simulink model "gdnn_lm_rtrl"  (R2017b)
settings: Solver=ode5  StartTime=0.0  StopTime=train_length  FixedStep=T_sim  RelTol=1e-3  EnableMultiTasking=on
values from neighbouring files (symbols this model uses):
  bb = zeros(1,numoflayers)    [ini_gdnn.m]
  bs = zeros(1,numoflayers)    [ini_gdnn.m]
  D_max = max(max(max(max(idel))),max(max(max(ldel))))    [ini_gdnn.m]
  DI_vec = [DI_vec DI(i,:)]    [ini_gdnn.m]
  DIB_vec = [DIB_vec DIB(i,:)]    [ini_gdnn.m]
  dimax = max(dimax)    [ini_gdnn.m]
  DIS_vec = [DIS_vec DIS(i,:)]    [ini_gdnn.m]
  DL_vec = [DL_vec DL(i,:)]    [ini_gdnn.m]
  DLB_vec = [DLB_vec DLB(i,:)]    [ini_gdnn.m]
  dlmax = max(dlmax)    [ini_gdnn.m]
  DLS_vec = [DLS_vec DLS(i,:)]    [ini_gdnn.m]
  E_LW_U = zeros(1,numoflayers^2)    [ini_gdnn.m]
  I = zeros(1,numoflayers*numofinputs)    [ini_gdnn.m]
  idelb_vec = 0    [ini_gdnn.m]
  idels_vec = 0    [ini_gdnn.m]
  Lb = zeros(1,numoflayers^2)    [ini_gdnn.m]
  ldelb_vec = 0    [ini_gdnn.m]
  ldels_vec = 0    [ini_gdnn.m]
  Lf = zeros(1,numoflayers^2)    [ini_gdnn.m]
  net_params = [Q, mue, theta, T, L, D_max, numoflayers, numofinputs, max(S), sum(R), S_out, S_target, print_weights, min_weights, prune_interval, train_length, prune_maxerr_OBS, prune_maxerr_exact]    [ini_gdnn.m]
  Q = 500    [ini_gdnn.m]
  T = 0.01    [APRBS_Anregung_APRBS.m]    (also in ini_gdnn.m)
  U = U_target    [ini_gdnn.m]
  U_out = zeros(1,numoflayers)    [ini_gdnn.m]
  U_target = zeros(1,numoflayers)    [ini_gdnn.m]
  W_alpha_ini = ones(1,L)    [ini_gdnn.m]
  W_ini = rand(1,L) - 0.5    [ini_gdnn.m]
  X = zeros(1,numoflayers)    [ini_gdnn.m]
undefined symbols (not defined in the file or in its folder): idel_vec, ldel_vec, R, S
libraries: mblibv1 x13, simulink x3
CloseFcn:
  | rtwprivate ssgencode ModelCloseRequest gdnn_lm_rtrl
settings Model: Creator=endisch  LastModifiedBy=Ussaema
settings DataIOCC: LimitDataPoints=on  SaveFormat=Array  SignalLoggingSaveFormat=ModelDataLogs
settings OptimizationCC: InitFltsAndDblsToZero=on  LifeSpan=inf
settings DebuggingCC: SaveWithParameterizedLinksMsg=none  UnderspecifiedInitializationDetection=Classic  MergeDetectMultiDrivingBlocksExec=none  SignalResolutionControl=TryResolveAllWithWarning  SolverPrmCheckMsg=warning  MultiTaskDSMMsg=warning  MultiTaskCondExecSysMsg=none  FcnCallInpInsideContextMsg=warning  StateNameClashWarn=warning  StrictBusMsg=None  SFUnexpectedBacktrackingDiag=warning  SFNoUnconditionalDefaultTransitionDiag=warning  SFExecutionAtInitializationDiag=none
settings HardwareCC: ProdBitPerPointer=32  ProdBitPerSizeT=32  ProdBitPerPtrDiffT=32  ProdLargestAtomicFloat=None  ProdIntDivRoundTo=Undefined  ProdEndianess=Unspecified  ProdWordSize=32  ProdHWDeviceType=32-bit Generic
settings ModelReferenceCC: PropagateSignalLabelsOutOfModel=off
settings CodeAppCC: StateflowObjectComments=on
settings GRTTargetCC: TargetFcnLib=ansi_tfl_tmw.mat  TargetLangStandard=C89/C90 (ANSI)  GeneratePreprocessorConditionals=Disable all  CombineOutputUpdateFcns=off  GRTInterface=on
settings ConfigComp: CovMetricSettings=dw  CovHtmlReporting=on  CovSaveCumulativeToWorkspaceVar=on  CovSaveSingleToWorkspaceVar=on  CovExternalEMLEnable=off

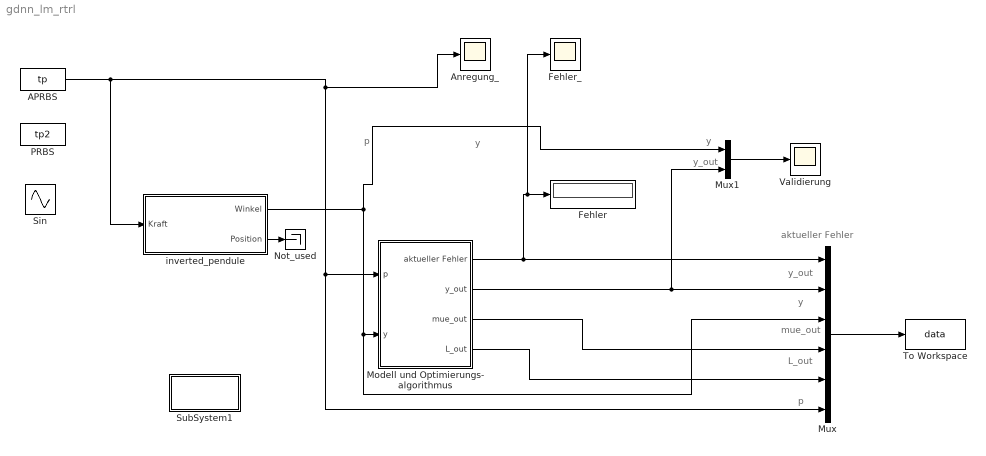
== system gdnn_lm_rtrl ==
  note: y_out
  note: y
  note: y
  note: p
  note: aktueller
      | Fehler
  note: y_out
  note: y
  note: mue_out
  note: L_out
  note: p
  APRBS : FromWorkspace  VariableName=tp  SampleTime=T  Interpolate=off  OutputAfterFinalValue=Cyclic repetition
  Anregung_ : Scope
  Fehler : Display
      settings: Format=short_e
  "Fehler_ " : Scope
  Modell und Optimierungs- algorithmus : Subsystem
  Mux : Mux  Inputs=6
  Mux1 : Mux  Inputs=2
  Not_used : Terminator
  PRBS : FromWorkspace  VariableName=tp2  SampleTime=T  Interpolate=off  OutputAfterFinalValue=Cyclic repetition
  Sin : Sin  Amplitude=5  Frequency=100  SampleTime=0
  SubSystem1 : Subsystem
      settings: OpenFcn=ini_gdnn
      mask Display: disp('Initialize\n(Double-Click)')
  To Workspace : ToWorkspace  VariableName=data  SaveFormat=Structure With Time  SampleTime=-1
  Validierung : Scope
  "inverted_pendule " : Subsystem  AncestorBlock=nichtlinearitaeten/Narendra Example 4
  wires:
  Mux/1 -> To Workspace/1
  "inverted_pendule "/1(Winkel) -> Mux1/1, Modell und Optimierungs- algorithmus/2(y), Mux/3
  APRBS/1 -> "inverted_pendule "/1(Kraft), Anregung_/1, Modell und Optimierungs- algorithmus/1(p), Mux/6
  Modell und Optimierungs- algorithmus/1(aktueller Fehler) -> "Fehler_ "/1, Fehler/1, Mux/1
  Modell und Optimierungs- algorithmus/3(mue_out) -> Mux/4
  Modell und Optimierungs- algorithmus/4(L_out) -> Mux/5
  Mux1/1 -> Validierung/1
  Modell und Optimierungs- algorithmus/2(y_out) -> Mux1/2, Mux/2
  "inverted_pendule "/2(Position) -> Not_used/1

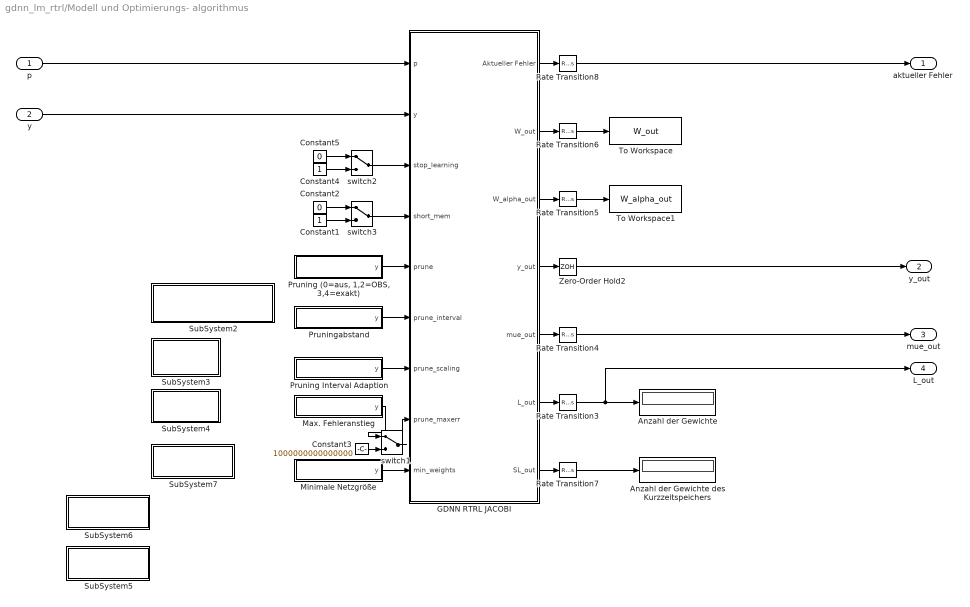
== system gdnn_lm_rtrl/Modell und Optimierungs- algorithmus ==
  p : Inport
  y : Inport  Port=2
  Anzahl der Gewichte : Display
  Anzahl der Gewichte des Kurzzeitspeichers : Display
  Constant1 : Constant
  Constant2 : Constant  Value=0
  Constant3 : Constant  Value=1000000000000000
  Constant4 : Constant
  Constant5 : Constant  Value=0
  GDNN RTRL JACOBI : Subsystem  TreatAsAtomicUnit=on  SystemSampleTime=T
  Max. Fehleranstieg : Subsystem  TreatAsAtomicUnit=on  SystemSampleTime=T  mask(Max. Error After Pruning-Step){number=10}
      mask prompts: number "Max. zulässig ist alter Fehler mal:"
      mask help: 0: Slider inaktiv, Wert wird aus der Ini-Datei (ini_gdnn.m) genommen
      mask Display: disp(sprintf('Fehleranstieg: %.1f',number));
  Minimale Netzgröße : Subsystem  TreatAsAtomicUnit=on  SystemSampleTime=T  mask(Minimum Number of Weights){number=1}
      mask prompts: number "Minimale Anzahl an Gewichte:"
      mask help: 0: Slider inaktiv, Wert wird aus der Ini-Datei (ini_gdnn.m) genommen
      mask Display: disp(sprintf('Gewichte: %i',number));
  "Pruning (0=aus, 1,2=OBS, 3,4=exakt)" : Subsystem  TreatAsAtomicUnit=on  SystemSampleTime=T  mask(Pruning Algorithms){number=0}
      mask prompts: number "Pruningverfahren:"
      mask help:
      | 0: aus
      | 1: OBS
      | 2: OBS, Berücksichtigung der Verzögerungsordnung
      | 3: exaktes Pruning
      | 4: exaktes Pruning, Berücksichtigung der Verzögerungsordnung
      mask TypeOptions number: 0 | 1 | 2 | 3 | 4
      mask Display: disp(sprintf('pruning %i',number-1));
  Pruning Interval Adaption : Subsystem  TreatAsAtomicUnit=on  SystemSampleTime=T  mask(Pruning Interval adaption){number=1}
      mask prompts: number "Skalierungsfaktor"
      mask help: 1.0: Pruning Interval wird nicht angepasst, Pruning Interval ist konstant
      mask Display: disp(sprintf('Scaling: %.1f',number));
  Pruningabstand : Subsystem  TreatAsAtomicUnit=on  SystemSampleTime=T  mask(Pruning Interval){number=100}
      mask prompts: number "Intervall (Abstand zweier Pruningschritte):"
      mask help: 0: Slider inaktiv, Wert wird aus der Ini-Datei (ini_gdnn.m) genommen
      mask Display: disp(sprintf('Intervall: %i',number));
  Rate Transition{3..8} (6 alike) : RateTransition  OutPortSampleTime=T
  SubSystem2 : Subsystem
      settings: OpenFcn=edit ini_gdnn.m gdnn_jacobi_rtrl.c forward_step.c get_jacobi_rtrl.c mem_alloc.c mem_free.c pruning_OBS.c w_conv.c transfer.c m_inv.c shift.c print_weights.c definitions.h;
      mask Display: disp('Load source files into editor\n(Double-Click)')
  SubSystem3 : Subsystem
      settings: OpenFcn="mex -v gdnn_jacobi_rtrl.c forward_step.c  get_jacobi_rtrl.c w_conv.c shift.c transfer.c m_inv.c pruning1_4.c mem_alloc.c mem_free.c print_weights.c"
      mask Display: disp('Mex files\n(Double-Click)')
  SubSystem4 : Subsystem
      settings: OpenFcn=clc
      mask Display: disp('Clear screen\n(Double-Click)')
  SubSystem5 : Subsystem
      settings: OpenFcn=|
      | net_params2 = net_params;
      | Q2=Q;
      | D_max2=D_max;
      | 
      | 
      | R2 = R;
      | S2 = S;
      | U2 = U;
      | X2 = X;
      | I2 = I;
      | Lf2 = Lf;
      | Lb2 = Lb;
      | E_LW_U2 = E_LW_U;
      | DI_vec2 = DI_vec;
      | DL_vec2 = DL_vec;
      | dimax2 = dimax;
      | dlmax2 = dlmax;
      | U_out2 = U_out;
      | U_target2 = U_target;
      | W_ini2 = W_out;
      | W_alpha_ini2 = W_alpha_out;
      | idel_vec2 = idel_vec;
      | ldel_vec2 = ldel_vec;
      | 
      | DIS_vec2=DIS_vec;
      | 
      | DLS_vec2=DLS_vec;
      | 
      | idels_vec2=idels_vec;
      | 
      | ldels_vec2=ldels_vec;
      | 
      | bs2=bs;
      | 
      | DIB_vec2=DIB_vec;
      | 
      | DLB_vec2=DLB_vec;
      | 
      | idelb_vec2=idelb_vec;
      | 
      | ldelb_vec2=ldelb_vec;
      | 
      | bb2= bb;
      | 
      | if exist('params.mat','file') ~= 0
      | !del params.mat
      | end
      | save params net_params2 Q2 D_max2 R2 S2 U2 X2 I2 Lf2 Lb2 E_LW_U2 DI_vec2 DL_vec2 dimax2 dlmax2 U_out2 U_target2 W_ini2 W_alpha_ini2 idel_vec2 ldel_vec2 DIS_vec2 DLS_vec2 idels_vec2 ldels_vec2 bs2 DIB_vec2 DLB_vec2 idelb_vec2 ldelb_vec2 bb2 ;
      | 
      | !copy params.mat ..\11.04.07Gesamtmodell\params.mat
      mask Display: disp('Create params.mat\n(Double-Click)')
  SubSystem6 : Subsystem
      settings: OpenFcn=save W W_out W_alpha_out;
      mask Display: disp('Save weights\n(Double-Click)')
  SubSystem7 : Subsystem
      settings: OpenFcn=|
      | load W;
      | W_ini=W_out;
      | W_alpha_ini=W_alpha_out;
      mask Display: disp('Load old weights\n(Double-Click)')
  To Workspace : ToWorkspace  VariableName=W_out  SampleTime=T
      settings: MaxDataPoints=1
  To Workspace1 : ToWorkspace  VariableName=W_alpha_out  SampleTime=T
      settings: MaxDataPoints=1
  Zero-Order Hold2 : ZeroOrderHold  SampleTime=T
  switch1 : ManualSwitch
  switch2 : ManualSwitch
  switch3 : ManualSwitch
  aktueller Fehler : Outport
  y_out : Outport  Port=2
  mue_out : Outport  Port=3
  L_out : Outport  Port=4
  wires:
  p/1 -> GDNN RTRL JACOBI/1(p)
  y/1 -> GDNN RTRL JACOBI/2(y)
  Constant4/1 -> switch2/2
  Rate Transition8/1 -> aktueller Fehler/1
  switch3/1 -> GDNN RTRL JACOBI/4(short_mem)
  GDNN RTRL JACOBI/4(y_out) -> Zero-Order Hold2/1
  "Pruning (0=aus, 1,2=OBS, 3,4=exakt)"/1(y) -> GDNN RTRL JACOBI/5(prune)
  Minimale Netzgröße/1(y) -> GDNN RTRL JACOBI/9(min_weights)
  Rate Transition7/1 -> Anzahl der Gewichte des Kurzzeitspeichers/1
  GDNN RTRL JACOBI/1(Aktueller Fehler) -> Rate Transition8/1
  GDNN RTRL JACOBI/6(L_out) -> Rate Transition3/1
  Pruning Interval Adaption/1(y) -> GDNN RTRL JACOBI/7("prune_scaling ")
  GDNN RTRL JACOBI/5(mue_out) -> Rate Transition4/1
  Constant2/1 -> switch3/1
  Rate Transition3/1 -> L_out/1, Anzahl der Gewichte/1
  Rate Transition5/1 -> To Workspace1/1
  Constant3/1 -> switch1/2
  GDNN RTRL JACOBI/3(W_alpha_out) -> Rate Transition5/1
  Rate Transition4/1 -> mue_out/1
  Constant5/1 -> switch2/1
  Constant1/1 -> switch3/2
  Zero-Order Hold2/1 -> y_out/1
  switch1/1 -> GDNN RTRL JACOBI/8(prune_maxerr)
  Rate Transition6/1 -> To Workspace/1
  Pruningabstand/1(y) -> GDNN RTRL JACOBI/6("prune_interval ")
  GDNN RTRL JACOBI/2(W_out) -> Rate Transition6/1
  GDNN RTRL JACOBI/7(SL_out) -> Rate Transition7/1
  Max. Fehleranstieg/1(y) -> switch1/1
  switch2/1 -> GDNN RTRL JACOBI/3(stop_learning)

== system gdnn_lm_rtrl/SubSystem1 ==

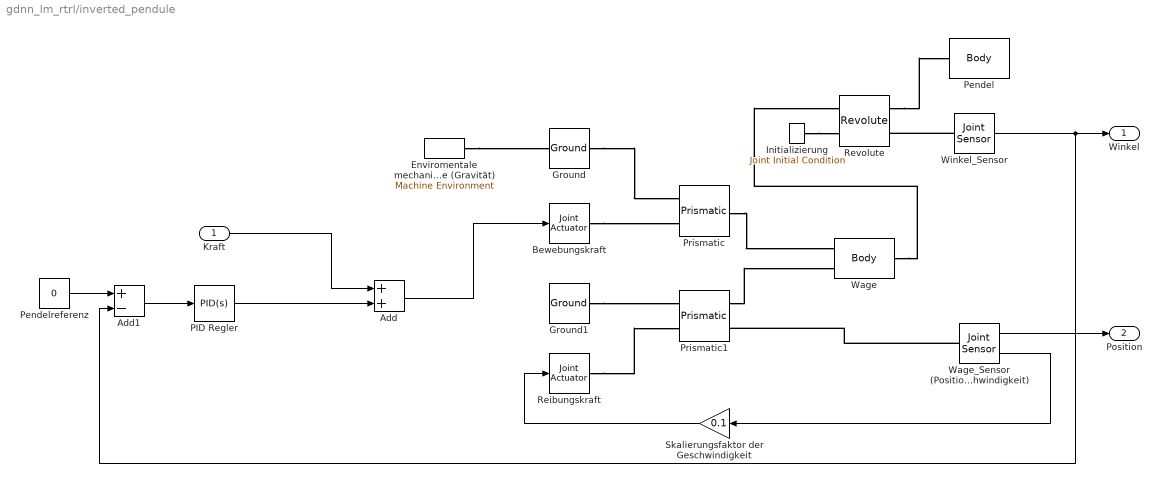
== system gdnn_lm_rtrl/inverted_pendule  ==
  Kraft : Inport
  Add : Sum
  Add1 : Sum  Inputs=+-
  Bewebungskraft : mblibv1/Sensors &  Actuators/Joint Actuator  UpdateFromCAD=off  PhysicalDomain=Mechanical  PortType=blob  ActuationStyle=Force  AngleUnits=deg  ArcVelocityUnits=deg/s  ArcAccelerationUnits=deg/s^2  CoordPositionUnits=m  VelocityUnits=m/s  AccelerationUnits=m/s^2  ForceUnits=N  TorqueUnits=N-m  ActiveIO=on  Width=1  DialogClass=MechanicalActuatorBlock  Primitive=P1  ReferenceFrame=Absolute (World)
      settings: SourceProductName=Simscape Multibody  SourceProductBaseCode=MS
  Enviromentale mechanische Zusammenhänge (Gravität) : mblibv1/Bodies/Machine Environment  PortType=env  PhysicalDomain=Mechanical  DialogTemplateClass=MECH.MachineEnvironment  SyncWhenCopied=off  Gravity=[0 -9.81 0]  GravityUnits=m/s^2  GravityAsSignal=off  Dimensionality=Auto-detect  AnalysisType=Forward dynamics  LinearAssemblyTolerance=1e-3  LinearAssemblyToleranceUnits=m  AngularAssemblyTolerance=1e-3  AngularAssemblyToleranceUnits=rad  ConstraintSolverType=Stabilizing  ConstraintRelTolerance=1e-4  ConstraintAbsTolerance=1e-4  UseRobustSingularityHandling=off  RedundancyAnalysisToleranceType=Automatically select tolerance  RedundancyAnalysisTolerance=1e-14  StatePerturbationType=Fixed  PerturbationSize=1e-5  VisualizeMachine=on  BodyVisualizationType=Use model default body geometries  BodyColorSelMode=Use model default  DefaultBodyColor=[1 0 0]
      settings: SourceProductName=Simscape Multibody  SourceProductBaseCode=MS
  Ground : mblibv1/Bodies/Ground  UpdateFromCAD=off  LeftPortType=env  RightPortType=workingframe  PhysicalDomain=Mechanical  DialogClass=GroundBlock  CoordPosition=[0 0 0]  CoordPositionUnits=m  StateVectorMgrId=0  MachineId=[1 0]  ShowEnvPort=on  ParameterChecksum=[3094704636, 429577838, 2456217209, 3197857456]  TopologyChecksum=[3735278374, 3704791383, 156068549, 4244875449]
      settings: SourceProductName=Simscape Multibody  SourceProductBaseCode=MS
  Ground1 : mblibv1/Bodies/Ground  UpdateFromCAD=off  LeftPortType=env  RightPortType=workingframe  PhysicalDomain=Mechanical  DialogClass=GroundBlock  CoordPosition=[0 0 0]  CoordPositionUnits=m  StateVectorMgrId=-1  MachineId=[0 0]  ShowEnvPort=off  ParameterChecksum=[0 0 0 0]  TopologyChecksum=[0 0 0 0]
      settings: SourceProductName=Simscape Multibody  SourceProductBaseCode=MS
  Initializierung : mblibv1/Sensors &  Actuators/Joint Initial Condition  UpdateFromCAD=off  LeftPortType=blob  RightPortType=blob  PhysicalDomain=mechanical  DialogClass=InitialConditionBlock  InitialConditions=P1$false$0$m$deg$0$m/s$deg/s#P2$false$0$m$deg$0$m/s$deg/s#P3$false$0$m$deg$0$m/s$deg/s#R1$true$0$m$deg$0$m/s$deg/s#R2$false$0$m$deg$0$m/s$deg/s#R3$false$0$m$deg$0$m/s$deg/s#S$false$0$m$deg$0$m/s$deg/s  P1PIC=0  P1VIC=0  P2PIC=0  P2VIC=0  P3PIC=0  P3VIC=0  R1PIC=0  R1VIC=0  R2PIC=0  R2VIC=0  R3PIC=0  R3VIC=0  SPIC=0  SVIC=0
      settings: SourceProductName=Simscape Multibody  SourceProductBaseCode=MS
  PID Regler : simulink/Continuous/PID Controller  Controller=PID  TimeDomain=Continuous-time  SampleTime=-1  IntegratorMethod=Forward Euler  FilterMethod=Forward Euler  Form=Parallel  UseFilter=on  ControllerParametersSource=internal  P=100  I=1  D=20  N=100  InitialConditionSource=internal  InitialConditionForIntegrator=0  InitialConditionForFilter=0  ExternalReset=none  LimitOutput=off  UpperSaturationLimit=inf  LowerSaturationLimit=-inf  LinearizeAsGain=on  AntiWindupMode=none  Kb=1  TrackingMode=off  Kt=1  PParamMin=[]  PParamMax=[]  IParamMin=[]  IParamMax=[]  DParamMin=[]  DParamMax=[]  NParamMin=[]  NParamMax=[]  KbParamMin=[]  KbParamMax=[]  KtParamMin=[]  KtParamMax=[]  POutMin=[]  POutMax=[]  IOutMin=[]  IOutMax=[]  DOutMin=[]  DOutMax=[]  NOutMin=[]  NOutMax=[]  KbOutMin=[]  KbOutMax=[]  KtOutMin=[]  KtOutMax=[]  IntegratorOutMin=[]  IntegratorOutMax=[]  FilterOutMin=[]  FilterOutMax=[]  SumOutMin=[]  SumOutMax=[]  SumI1OutMin=[]  SumI1OutMax=[]  SumI2OutMin=[]  SumI2OutMax=[]  SumI3OutMin=[]  SumI3OutMax=[]  SumDOutMin=[]  SumDOutMax=[]  SaturationOutMin=[]  SaturationOutMax=[]  IntegratorContinuousStateAttributes=''  IntegratorStateMustResolveToSignalObject=off  IntegratorRTWStateStorageClass=Auto  FilterContinuousStateAttributes=''  FilterStateMustResolveToSignalObject=off  FilterRTWStateStorageClass=Auto  DifferentiatorICPrevScaledInput=0  DifferentiatorOutMin=[]  DifferentiatorOutMax=[]  InitialConditionSetting=State (most efficient)  FilterDiffOutCoefMin=[]  FilterDiffOutCoefMax=[]  SumDenOutMin=[]  SumDenOutMax=[]  SumNumOutMin=[]  SumNumOutMax=[]  ReciprocalOutMin=[]  ReciprocalOutMax=[]  DivideOutMin=[]  DivideOutMax=[]  TunerSelectOption=Transfer Function Based (PID Tuner App)
  Pendel : mblibv1/Bodies/Body  LConnTagsString=CS1  UpdateFromCAD=off  DialogClass=MechanicalBodyBlock  Mass=0.2  MassUnits=kg  InertiaUnits=kg*m^2  Inertia=0.006*eye(3)  Shape=Cylinder  ShapeDims=[1 1]  ShapeUnits=m  ShapeUse=false  Density=1  DensityUnits=kg/m^3  DensityUse=false  GraphicsMode=MACHINE_DEFAULT  BodyColorSelMode=MACHINE_DEFAULT  BodyColor=[1 0 0]  AttachedToCS=CG  CG=Left$CG$[0 0.3 0]$CS1$CS1$m$[0 0 0]$Euler X-Y-Z$deg$WORLD$false$none  WorkingFrames=Left$CS1$[0 0 0]$Adjoining$Adjoining$m$[0 0 0]$Euler X-Y-Z$deg$WORLD$true$none#Right$CS2$[0.1 0 0]$CS1$CS1$m$[0 0 0]$Euler X-Y-Z$deg$WORLD$false$none#Right$CS3$[-0.1 0 0]$CS1$CS1$m$[0 0 0]$Euler X-Y-Z$deg$WORLD$false$none#Right$CS4$[-0.1 0.6 0]$CS1$CS1$m$[0 0 0]$Euler X-Y-Z$deg$WORLD$false$none#Right$CS5$[0.1 0.6 0]$CS1$CS1$m$[0 0 0]$Euler X-Y-Z$deg$WORLD$false$none  CGPos=[0 0.3 0]  CGRot=[0 0 0]  CS0Pos=[]  CS0Rot=[]  CS1Pos=[0 0 0]  CS1Rot=[0 0 0]  CS2Pos=[0.1 0 0]  CS2Rot=[0 0 0]  CS3Pos=[-0.1 0 0]  CS3Rot=[0 0 0]  CS4Pos=[-0.1 0.6 0]  CS4Rot=[0 0 0]  CS5Pos=[0.1 0.6 0]  CS5Rot=[0 0 0]  CS6Pos=[]  CS6Rot=[]  CS7Pos=[]  CS7Rot=[]  CS8Pos=[]  CS8Rot=[]  CS9Pos=[]  CS9Rot=[]  CS10Pos=[]  CS10Rot=[]  CS11Pos=[]  CS11Rot=[]  CS12Pos=[]  CS12Rot=[]  CS13Pos=[]  CS13Rot=[]  CS14Pos=[]  CS14Rot=[]  CS15Pos=[]  CS15Rot=[]  CS16Pos=[]  CS16Rot=[]  CS17Pos=[]  CS17Rot=[]  CS18Pos=[]  CS18Rot=[]  CS19Pos=[]  CS19Rot=[]  CS20Pos=[]  CS20Rot=[]
      settings: SourceProductName=Simscape Multibody  SourceProductBaseCode=MS
  Pendelreferenz : Constant  Value=0
  Prismatic : mblibv1/Joints/Prismatic  LConnTagsString=__newl0|SA1  RConnTagsString=__newr0  UpdateFromCAD=off  NumSAPorts=1  CutJoint=off  MarkAsCut=off  Primitives=prismatic  PrimitiveProps=P1$World$[1 0 0]$prismatic  DialogClass=JointBlock  P1Axis=[1 0 0]
      settings: SourceProductName=Simscape Multibody  SourceProductBaseCode=MS
  Prismatic1 : mblibv1/Joints/Prismatic  LConnTagsString=__newl0|SA1  RConnTagsString=__newr0|SA1  UpdateFromCAD=off  NumSAPorts=2  CutJoint=off  MarkAsCut=off  Primitives=prismatic  PrimitiveProps=P1$World$[1 0 0]$prismatic  DialogClass=JointBlock  P1Axis=[1 0 0]
      settings: SourceProductName=Simscape Multibody  SourceProductBaseCode=MS
  Reibungskraft : mblibv1/Sensors &  Actuators/Joint Actuator  UpdateFromCAD=off  PhysicalDomain=Mechanical  PortType=blob  ActuationStyle=Force  AngleUnits=deg  ArcVelocityUnits=deg/s  ArcAccelerationUnits=deg/s^2  CoordPositionUnits=m  VelocityUnits=m/s  AccelerationUnits=m/s^2  ForceUnits=N  TorqueUnits=N-m  ActiveIO=on  Width=1  DialogClass=MechanicalActuatorBlock  Primitive=P1  ReferenceFrame=Absolute (World)
      settings: SourceProductName=Simscape Multibody  SourceProductBaseCode=MS
  Revolute : mblibv1/Joints/Revolute  LConnTagsString=__newl0|SA1  RConnTagsString=__newr0|SA1  UpdateFromCAD=off  NumSAPorts=2  CutJoint=off  MarkAsCut=off  Primitives=prismatic  PrimitiveProps=R1$World$[0 0 1]$revolute  DialogClass=JointBlock  R1Axis=[0 0 1]
      settings: SourceProductName=Simscape Multibody  SourceProductBaseCode=MS
  Skalierungsfaktor der Geschwindigkeit : Gain  Gain=0.1
  Wage : mblibv1/Bodies/Body  LConnTagsString=CS1|CS2  RConnTagsString=CS3  UpdateFromCAD=off  DialogClass=MechanicalBodyBlock  Mass=5  MassUnits=kg  InertiaUnits=kg*m^2  Inertia=eye(3)  Shape=Cylinder  ShapeDims=[1 1]  ShapeUnits=m  ShapeUse=false  Density=1  DensityUnits=kg/m^3  DensityUse=false  GraphicsMode=MACHINE_DEFAULT  BodyColorSelMode=MACHINE_DEFAULT  BodyColor=[1 0 0]  AttachedToCS=CG  CG=Left$CG$[0 0 0]$WORLD$WORLD$m$[0 0 0]$Euler X-Y-Z$deg$WORLD$false$none  WorkingFrames=Left$CS1$[-1 0 0]$CG$CG$m$[0 0 0]$Euler X-Y-Z$deg$WORLD$true$none#Left$CS2$[0 0 0]$CG$CG$m$[0 0 0]$Euler X-Y-Z$deg$WORLD$true$none#Right$CS3$[0 0.5 0]$CG$CG$m$[0 0 0]$Euler X-Y-Z$deg$WORLD$true$none#Right$CS4$[-1 0.5 0]$CG$CG$m$[0 0 0]$Euler X-Y-Z$deg$WORLD$false$none#Right$CS5$[-1 -0.5 0]$CG$CG$m$[0 0 0]$Euler X-Y-Z$deg$WORLD$false$none#Right$CS6$[1 -0.5 0]$CG$CG$m$[0 0 0]$Euler X-Y-Z$deg$WORLD$false$none#Right$CS7$[1 0.5 0]$CG$CG$m$[0 0 0]$Euler X-Y-Z$deg$WORLD$false$none  CGPos=[0 0 0]  CGRot=[0 0 0]  CS0Pos=[]  CS0Rot=[]  CS1Pos=[-1 0 0]  CS1Rot=[0 0 0]  CS2Pos=[0 0 0]  CS2Rot=[0 0 0]  CS3Pos=[0 0.5 0]  CS3Rot=[0 0 0]  CS4Pos=[-1 0.5 0]  CS4Rot=[0 0 0]  CS5Pos=[-1 -0.5 0]  CS5Rot=[0 0 0]  CS6Pos=[1 -0.5 0]  CS6Rot=[0 0 0]  CS7Pos=[1 0.5 0]  CS7Rot=[0 0 0]  CS8Pos=[]  CS8Rot=[]  CS9Pos=[]  CS9Rot=[]  CS10Pos=[]  CS10Rot=[]  CS11Pos=[]  CS11Rot=[]  CS12Pos=[]  CS12Rot=[]  CS13Pos=[]  CS13Rot=[]  CS14Pos=[]  CS14Rot=[]  CS15Pos=[]  CS15Rot=[]  CS16Pos=[]  CS16Rot=[]  CS17Pos=[]  CS17Rot=[]  CS18Pos=[]  CS18Rot=[]  CS19Pos=[]  CS19Rot=[]  CS20Pos=[]  CS20Rot=[]
      settings: SourceProductName=Simscape Multibody  SourceProductBaseCode=MS
  "Wage_Sensor (Position, Geschwindigkeit)" : mblibv1/Sensors &  Actuators/Joint Sensor  UpdateFromCAD=off  PhysicalDomain=Mechanical  PortType=blob  Muxed=off  Pose=off  Angle=on  AngleUnits=deg  ArcVelocity=off  ArcVelocityUnits=deg/s  ArcAcceleration=off  ArcAccelerationUnits=deg/s^2  CoordPosition=on  CoordPositionUnits=m  Velocity=on  VelocityUnits=m/s  Acceleration=off  AccelerationUnits=m/s^2  Quaternion=on  QuaternionDT=off  QuaternionDDT=off  QuaternionUnits=off  OutputVector=[1]  ActiveIO=on  Width=2  DialogClass=MechanicalSensorBlock  Primitive=P1  Force=off  ForceUnits=N  Torque=off  TorqueUnits=N*m  ReferenceFrame=Absolute (World)  ReactionSensedSide=Base  ReactionReferenceFrame=Absolute (World)  ReactionForce=off  ReactionForceUnits=N  ReactionMoment=off  ReactionMomentUnits=N*m
      settings: SourceProductName=Simscape Multibody  SourceProductBaseCode=MS
  Winkel_Sensor : mblibv1/Sensors &  Actuators/Joint Sensor  UpdateFromCAD=off  PhysicalDomain=Mechanical  PortType=blob  Muxed=on  Pose=off  Angle=on  AngleUnits=rad  ArcVelocity=off  ArcVelocityUnits=deg/s  ArcAcceleration=off  ArcAccelerationUnits=deg/s^2  CoordPosition=on  CoordPositionUnits=m  Velocity=off  VelocityUnits=m/s  Acceleration=off  AccelerationUnits=m/s^2  Quaternion=on  QuaternionDT=off  QuaternionDDT=off  QuaternionUnits=off  OutputVector=[1]  ActiveIO=on  Width=1  DialogClass=MechanicalSensorBlock  Primitive=R1  Force=off  ForceUnits=N  Torque=off  TorqueUnits=N*m  ReferenceFrame=Absolute (World)  ReactionSensedSide=Base  ReactionReferenceFrame=Absolute (World)  ReactionForce=off  ReactionForceUnits=N  ReactionMoment=off  ReactionMomentUnits=N*m
      settings: SourceProductName=Simscape Multibody  SourceProductBaseCode=MS
  Winkel : Outport
  Position : Outport  Port=2
  wires:
  PID Regler/1 -> Add/2
  Add1/1 -> PID Regler/1
  Kraft/1 -> Add/1
  Pendelreferenz/1 -> Add1/1
  Winkel_Sensor/1 -> Add1/2, Winkel/1
  Skalierungsfaktor der Geschwindigkeit/1 -> Reibungskraft/1
  "Wage_Sensor (Position, Geschwindigkeit)"/2 -> Skalierungsfaktor der Geschwindigkeit/1
  Add/1 -> Bewebungskraft/1
  "Wage_Sensor (Position, Geschwindigkeit)"/1 -> Position/1
  connections:
  Bewebungskraft/RConn1 -- Prismatic/LConn2
  Initializierung/RConn1 -- Revolute/LConn2
  Reibungskraft/RConn1 -- Prismatic1/LConn2
  Ground/RConn1 -- Prismatic/LConn1
  "Wage_Sensor (Position, Geschwindigkeit)"/LConn1 -- Prismatic1/RConn2
  Enviromentale mechanische Zusammenhänge (Gravität)/RConn1 -- Ground/LConn1
  Ground1/RConn1 -- Prismatic1/LConn1
  Wage/RConn1 -- Revolute/LConn1
  Prismatic1/RConn1 -- Wage/LConn2
  Prismatic/RConn1 -- Wage/LConn1
  Winkel_Sensor/LConn1 -- Revolute/RConn2
  Revolute/RConn1 -- Pendel/LConn1

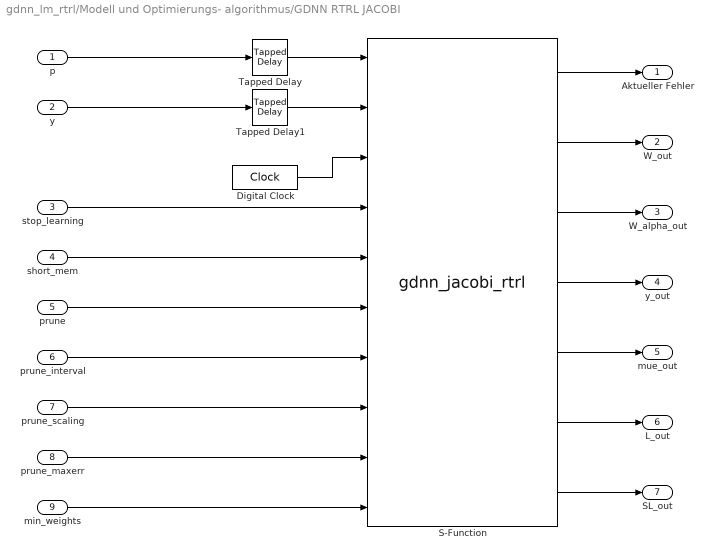
== system gdnn_lm_rtrl/Modell und Optimierungs- algorithmus/GDNN RTRL JACOBI ==
  p : Inport
  y : Inport  Port=2
  stop_learning : Inport  Port=3
  short_mem : Inport  Port=4
  prune : Inport  Port=5
  "prune_interval " : Inport  Port=6
  "prune_scaling " : Inport  Port=7
  prune_maxerr : Inport  Port=8
  min_weights : Inport  Port=9
  Digital Clock : DigitalClock  SampleTime=T
  S-Function : S-Function  FunctionName=gdnn_jacobi_rtrl  Parameters=net_params,R,S,U,X,I,Lf,Lb,E_LW_U,DI_vec,DL_vec,dimax,dlmax,U_out,U_target,W_ini,W_alpha_ini,idel_vec,ldel_vec,DIS_vec,DLS_vec,idels_vec,ldels_vec,bs,DIB_vec,DLB_vec,idelb_vec,ldelb_vec,bb  SFunctionModules=forward_step.c get_jacobi_rtrl.c w_conv.c shift.c transfer.c m_inv.c pruning1_4.c mem_alloc.c mem_free.c  SFunctionDeploymentMode=off  EnableBusSupport=off
  Tapped Delay : simulink/Discrete/Tapped Delay  vinit=0.0  samptime=-1  NumDelays=Q+D_max-1  DelayOrder=Oldest  includeCurrent=on
  Tapped Delay1 : simulink/Discrete/Tapped Delay  vinit=0.0  samptime=-1  NumDelays=Q-1  DelayOrder=Oldest  includeCurrent=on
  Aktueller Fehler : Outport
  W_out : Outport  Port=2
  W_alpha_out : Outport  Port=3
  y_out : Outport  Port=4
  mue_out : Outport  Port=5
  L_out : Outport  Port=6
  SL_out : Outport  Port=7
  wires:
  Digital Clock/1 -> S-Function/3
  S-Function/1 -> Aktueller Fehler/1
  S-Function/2 -> W_out/1
  S-Function/3 -> W_alpha_out/1
  S-Function/4 -> y_out/1
  S-Function/5 -> mue_out/1
  S-Function/6 -> L_out/1
  S-Function/7 -> SL_out/1
  stop_learning/1 -> S-Function/4
  short_mem/1 -> S-Function/5
  prune/1 -> S-Function/6
  "prune_interval "/1 -> S-Function/7
  "prune_scaling "/1 -> S-Function/8
  prune_maxerr/1 -> S-Function/9
  min_weights/1 -> S-Function/10
  y/1 -> Tapped Delay1/1
  Tapped Delay/1 -> S-Function/1
  Tapped Delay1/1 -> S-Function/2
  p/1 -> Tapped Delay/1

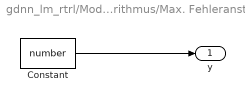
== system gdnn_lm_rtrl/Modell und Optimierungs- algorithmus/Max. Fehleranstieg ==
  Constant : Constant  Value=number
  y : Outport
  wires:
  Constant/1 -> y/1

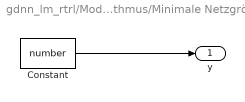
== system gdnn_lm_rtrl/Modell und Optimierungs- algorithmus/Minimale Netzgröße ==
  Constant : Constant  Value=number
  y : Outport
  wires:
  Constant/1 -> y/1

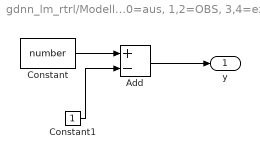
== system gdnn_lm_rtrl/Modell und Optimierungs- algorithmus/Pruning (0=aus, 1,2=OBS, 3,4=exakt) ==
  Add : Sum  Inputs=+-
  Constant : Constant  Value=number
  Constant1 : Constant
  y : Outport
  wires:
  Constant/1 -> Add/1
  Add/1 -> y/1
  Constant1/1 -> Add/2

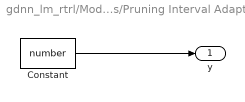
== system gdnn_lm_rtrl/Modell und Optimierungs- algorithmus/Pruning Interval Adaption ==
  Constant : Constant  Value=number
  y : Outport
  wires:
  Constant/1 -> y/1

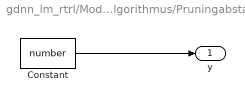
== system gdnn_lm_rtrl/Modell und Optimierungs- algorithmus/Pruningabstand ==
  Constant : Constant  Value=number
  y : Outport
  wires:
  Constant/1 -> y/1

== system gdnn_lm_rtrl/Modell und Optimierungs- algorithmus/SubSystem2 ==

== system gdnn_lm_rtrl/Modell und Optimierungs- algorithmus/SubSystem3 ==

== system gdnn_lm_rtrl/Modell und Optimierungs- algorithmus/SubSystem4 ==

== system gdnn_lm_rtrl/Modell und Optimierungs- algorithmus/SubSystem5 ==

== system gdnn_lm_rtrl/Modell und Optimierungs- algorithmus/SubSystem6 ==

== system gdnn_lm_rtrl/Modell und Optimierungs- algorithmus/SubSystem7 ==
